simulink model "MPC_with_PI"  (R2021b)
settings: Solver=VariableStepAuto  StartTime=0.0  StopTime=115  FixedStep=0.1  RelTol=1e-2
InitFcn:
  | clear all;
  | 
  | 
  | %Path in global coordinate reference frame - X and Y
  | 
  | xRef=[
  | 57.222
  | 52.707
  | 48.874
  | 44.359
  | 39.930
  | 35.160
  | 31.071
  | 16.591
  | 7.391
  | -2.575
  | -9.901
  | -13.563
  | -16.289
  | -17.567
  | -15.437
  | -8.538
  | -2.745
  | 1.002
  | 6.624
  | 10.628
  | 15.654
  | 20.935
  | 24.853
  | 28.260
  | 31.327
  | 33.797
  | 35.841
  | 36.182
  | 35.671
  | 34.478
  | 32.008
  | 29.964
  | 28.005
  | 26.301
  | 25.109
  | 24.001
  | 23.149
  | 22.383
  | 21.957
  | 21.531
  | 21.190
  | 20.850
  | 20.594
  | 21.105
  | 21.531
  | 21.701
  | 21.701
  | 21.531
  | 21.361
  | 21.446
  | 22.042
  | 23.831
  | 25.875
  | 28.771
  | 35.245
  | 41.208
  | 49.130
  | 53.814
  | 58.585
  | 64.377
  | 71.021
  | 79.113
  | 86.439
  | 94.360
  | 100.153
  | 103.304
  | 105.400
  | 105.989
  | 105.989
  | 105.989
  | 105.989
  | 105.989
  | 106.540
  | 107.393
  | 107.904
  | 108.500
  | 109.267
  | 109.948
  | 110.204
  | 110.204
  | 110.204
  | 110.289
  | 110.204
  | 110.204
  | 110.034
  | 109.608
  | 108.500
  | 107.393
  | 106.456
  | 105.775
  | 105.775
  | 105.689
  | 105.689
  | 105.775
  | 105.689
  | 105.775
  | 105.775
  | 105.604];
  | 
  | 
  | yRef=[65.95708466
  | 66.72370911
  | 67.31997681
  | 68.17178345
  | 68.9384079
  | 69.79021454
  | 70.55683899
  | 72.43080902
  | 73.1974411
  | 73.02707672
  | 70.98274231
  | 69.44949341
  | 67.06443787
  | 63.40166855
  | 57.3538475
  | 52.15782928
  | 45.76928711
  | 39.21038055
  | 32.82183456
  | 29.92569351
  | 27.71099854
  | 26.09256744
  | 24.38895607
  | 22.42980194
  | 19.27812004
  | 16.21161842
  | 11.95258808
  | 7.182474136
  | 2.412360907
  | -1.676307797
  | -5.679795742
  | -9.257381439
  | -12.74978542
  | -16.66809273
  | -19.81977463
  | -23.05663872
  | -26.37868118
  | -30.21180725
  | -33.53385162
  | -36.855896
  | -40.34830093
  | -43.75552368
  | -49.03672028
  | -58.32140732
  | -65.81729889
  | -81.49052429
  | -89.32714081
  | -106.0225372
  | -109.0890427
  | -111.8148193
  | -114.6257782
  | -116.2
  | -116.4997559
  | -116.4997559
  | -116.4997559
  | -116.4997559
  | -116.4997559
  | -116.4997559
  | -116.4997559
  | -116.4997559
  | -116.4997559
  | -116.4997559
  | -116.0738525
  | -116.0738525
  | -116.0738525
  | -115.7331314
  | -114.7961426
  | -113.1777115
  | -110.7074738
  | -106.7039871
  | -99.20809174
  | -92.47882843
  | -87.19763184
  | -85.40883636
  | -83.70522308
  | -82.17197418
  | -80.63872528
  | -78.25366211
  | -75.35752869
  | -71.86511993
  | -63.94332504
  | -56.95851517
  | -51.16623688
  | -45.20359421
  | -42.90371704
  | -40.26311874
  | -37.62252045
  | -35.2374649
  | -33.19313049
  | -30.63771057
  | -27.91193199
  | -25.35651398
  | -19.73459435
  | -13.51641083
  | -7.29822731
  | -1.505946636
  | 3.775250435
  | 19.87438393];
  | 
  | %initial positions for the car
  | X_o=57.22167206;
  | Y_o=65.95708466;
  | psi_o=2.971793445;
  | 
  | %Useless code, used for plotter XY block.
  | s = size(xRef);
  | Ts=str2double(get_param(gcs, 'StopTime'));
  | tRef = (linspace(0,Ts,s(1)))';
libraries: autolibutils x4, autolibshared x2, sim3dlib x2, vehdynlibviscommon x1, slpidlib x1, simulink x1, vdynlib x1, vehdynlibsteering x1, eeGeneralControl x1, dspvision x1
(part 1 of 3)
settings Model: Creator=tapan  LastModifiedBy=tapan
settings SolverCC: ZeroCrossAlgorithm=Adaptive

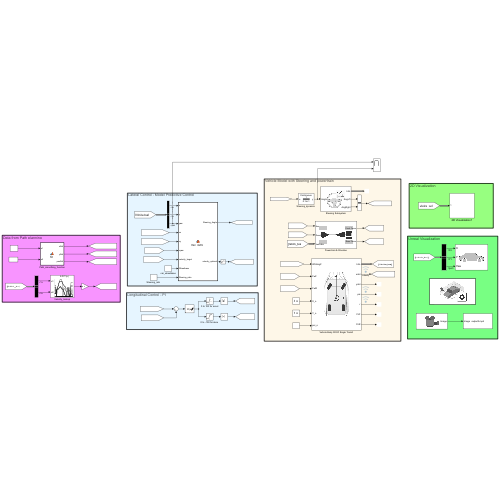
[thumbnail: Simulink's stored preview of the top-level diagram]
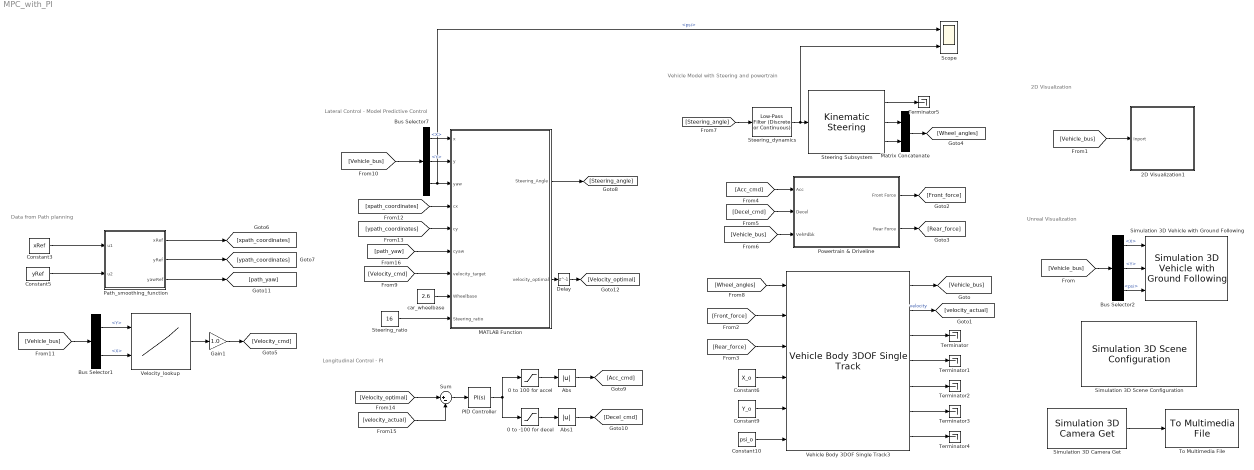
== system MPC_with_PI ==
  note: Data from Path planning
  note: Longitudinal Control - PI
  note: Vehicle Model with Steering and powertrain
  note: Unreal Visualization
  note: 2D Visualization
  note: Lateral Control - Model Predictive Control
  0 to -100 for decel : Saturate  UpperLimit=0  LowerLimit=-100
  0 to 100 for accel : Saturate  UpperLimit=100  LowerLimit=0
  2D Visualization1 : Subsystem
  Abs : Abs
  Abs1 : Abs
  Bus Selector1 : BusSelector  OutputSignals=InertFrm.Cg.Disp.Y,InertFrm.Cg.Disp.X
  Bus Selector2 : BusSelector  OutputSignals=InertFrm.Cg.Disp.X,InertFrm.Cg.Disp.Y,InertFrm.Cg.Ang.psi
  Bus Selector7 : BusSelector  OutputSignals=InertFrm.Cg.Disp.X,InertFrm.Cg.Disp.Y,InertFrm.Cg.Ang.psi
  Constant10 : Constant  Value=psi_o
  Constant3 : Constant  Value=xRef  SampleTime=0.1
  Constant5 : Constant  Value=yRef  SampleTime=0.1
  Constant6 : Constant  Value=X_o
  Constant9 : Constant  Value=Y_o
  Delay : Delay  DelayLength=1  InitialCondition=0
  Gain1 : Gain  Gain=1.0
  MATLAB Function : MATLAB Function
  Matrix Concatenate : Concatenate
  PID Controller : slpidlib/PID Controller  Controller=PI  Form=Parallel  TimeDomain=Continuous-time  UseExternalTs=off  SampleTime=-1  IntegratorMethod=Forward Euler  FilterMethod=Forward Euler  ControllerParametersSource=internal  P=1  I=5  D=0  UseFilter=on  N=100  TunerSelectOption=Transfer Function Based (PID Tuner App)  InitialConditionSource=internal  InitialConditionForIntegrator=0  InitialConditionForFilter=0  DifferentiatorICPrevScaledInput=0  ExternalReset=none  TrackingMode=off  Kt=1  LimitOutput=on  SatLimitsSource=internal  UpperSaturationLimit=100  LowerSaturationLimit=-100  LinearizeAsGain=on  AntiWindupMode=clamping  Kb=1  POutMin=[]  POutMax=[]  IOutMin=[]  IOutMax=[]  DOutMin=[]  DOutMax=[]  NOutMin=[]  NOutMax=[]  SumOutMin=[]  SumOutMax=[]  SaturationOutMin=[]  SaturationOutMax=[]  PParamMin=[]  PParamMax=[]  IParamMin=[]  IParamMax=[]  DParamMin=[]  DParamMax=[]  NParamMin=[]  NParamMax=[]  KbParamMin=[]  KbParamMax=[]  KtParamMin=[]  KtParamMax=[]  KbOutMin=[]  KbOutMax=[]  KtOutMin=[]  KtOutMax=[]  IntegratorOutMin=[]  IntegratorOutMax=[]  FilterOutMin=[]  FilterOutMax=[]  SumI1OutMin=[]  SumI1OutMax=[]  SumI2OutMin=[]  SumI2OutMax=[]  SumI3OutMin=[]  SumI3OutMax=[]  SumI4OutMin=[]  SumI4OutMax=[]  SumDOutMin=[]  SumDOutMax=[]  DifferentiatorOutMin=[]  DifferentiatorOutMax=[]  FilterDiffOutCoefMin=[]  FilterDiffOutCoefMax=[]  ReciprocalOutMin=[]  ReciprocalOutMax=[]  SumDenOutMin=[]  SumDenOutMax=[]  SumNumOutMin=[]  SumNumOutMax=[]  DivideOutMin=[]  DivideOutMax=[]  UdiffTsProdOutMin=[]  UdiffTsProdOutMax=[]  NTsProdOutMin=[]  NTsProdOutMax=[]  UintegralTsProdOutMin=[]  UintegralTsProdOutMax=[]  UngainTsProdOutMin=[]  UngainTsProdOutMax=[]  IntegratorContinuousStateAttributes=''  IntegratorStateMustResolveToSignalObject=off  IntegratorRTWStateStorageClass=Auto  FilterContinuousStateAttributes=''  FilterStateMustResolveToSignalObject=off  FilterRTWStateStorageClass=Auto  ParallelPVariant=InternalParameters  IdealPVariant=Disabled  IVariant=InternalParameters  DVariant=Disabled  IntegratorVariant=Continuous  SatVariant=Enabled  AWVariant=ContClampingParallel  PCopyVariant=Disabled  TRVariant=Disabled  FdbkBlocksVariant=Forward  IdealPFdbkVariant=Disabled  SatFdbkVariant=Disabled  DerivativeFilterVariant=Disabled  NVariant=Disabled  NCopyVariant=Disabled_SignalSpec  FilterICVariant=Disabled  IntegratorICVariant=InternalICs  ExternalResetVariant=Disabled  TRSumVariant=Passthrough  SumFdbkVariant=Disabled  SumVariant=Sum_PI  TsampFilterVariant=InternalTs  TsampNgainVariant=Passthrough  TsampIntegralVariant=Passthrough  ExternalSaturationOutDataTypeStr=Inherit: Same as second input
  Path_smoothing_function : MATLAB Function  TreatAsAtomicUnit=on
  Powertrain & Driveline : Subsystem
      mask Display: image('vdbslibpt.png');
  Scope : Scope  NumInputPorts=2
  Simulation 3D Camera Get : sim3dlib/Simulation 3D Camera Get  Priority=1  sensorTag=Sim3dSensor1  sensorId=1  sensorName=Sim3dSensor1  vehTagList={'Scene Origin';'SimulinkVehicle1'}  vehTag=SimulinkVehicle1  mountLoc=Hood center  offsetFlag=on  tmountOffset=[-10, 0, 7]  rmountOffset=[0, 25, 0]  HorizontalResolution=1280  VerticalResolution=720  HorizontalFOV=120  SampleTime=-1  mountPoint=[-8.53600025177002 0 8.10000038146973]  mountOrientation=[0 -25 0]  aMode=2  ID=1
      settings: SourceProductBaseCode=AE,DR,UV,VE
  Simulation 3D Scene Configuration : sim3dlib/Simulation 3D Scene Configuration  Priority=0  ProjectFormat_internal=Default Scenes  ProjectFormat=Default Scenes  SceneDesc=Virtual Mcity  ProjectName=C:\Program Files\MATLAB\R2021b\toolbox\shared\sim3d_projects\automotive_project\UE4\WindowsNoEditor\VehicleSimulation.exe  ScenePath=/Game/Maps/HwStrght  vehTagList={'Scene Origin';'SimulinkVehicle1'}  vehTag=SimulinkVehicle1  OpVisEn=off  Ts=0.05  EnableWindow=off  EnableWeather=off  SunAltitude=40.0  SunAzimuth=90  clouds=10  wind=1  fog=0  rain=0  sensorTag=MainCamera1  sensorId=1  sensorName=MainCamera1  mountLoc=Origin  offsetFlag=off  tmountOffset=[0, 0, 0]  rmountOffset=[0, 0, 0]  HorizontalResolution=1280  VerticalResolution=720  HorizontalFOV=60  mountPoint=[0 0 0]  mountOrientation=[0 0 0]  aMode=3  ID=1
      settings: SourceProductBaseCode=AE,DR,UV,VE
  Simulation 3D Vehicle with Ground Following : vdynlib/Vehicle Scenarios/Sim3D/Sim3D Vehicle/Components/Simulation 3D Vehicle with Ground Following  Priority=-1  PassVehMesh=Sedan  PassVehMesh_Internal=Sedan  MeshPath=/MathWorksSimulation/Vehicles/Muscle/Meshes/SK_MuscleCar.SK_MuscleCar  TrackWidth=1.9  WheelBase=3  WheelRadius=0.35  VehColor=Silver  VehColor_Internal=Silver  InitialPos=[0, 0, 0]  InitialRot=[0, 0, 0]  ActorName=SimulinkVehicle1  VehLightsControl=off  HeadlightColor=[ 1, 1, 1 ]  HighBeamIntensity=100000  LowBeamIntensity=60000  HighBeamConeAngle=1.22  LowBeamConeAngle=1.22  LeftHeadlightOrientation=[ 0, 0 ]  RightHeadlightOrientation=[ 0, 0 ]  BrakelightIntensity=200  ReverselightIntensity=500  SignallightIntensity=500  SignallightPeriod=1  SignalPulseWidth=50  SampleTime=-1  ActorType=SimulinkVehicle  ID=1  aMode=2  ActorTag=SimulinkVehicle1  CoordinateScheme=SAE
      settings: SourceProductBaseCode=VE
  Steering Subsystem : vehdynlibsteering/Kinematic Steering  StrgType=Ackerman  StrgRatioType=Constant  Loc=Front  NrmlFctr=0.01  TrckWdth=1.4  WhlBase=2.6  Db=0  StrgRng=5*pi  StrgAngBpts="[-6.2832   -5.0265   -3.7699   -2.5133   -1.2566         0    1.2566    2.5133    3.7699    5.0265    6.2832]"  StrgRatioTbl=|  StrgRatio=16  StrgArmLngth=0.1  RckCsLngth=0.5  TieRodLngth=0.248  D=0.2  PnnRadius=0.0057  PnnRadiusTbl="[0.0055    0.0055    0.0056    0.0057    0.0058    0.0057    0.0057    0.0057    0.0056    0.0055    0.0055]"  RodLngth=0.1  ParaArmLngth=0.9  aMode=2
      | [13.5000   13.3750   13.2500   13.1250   13.0000   13.0000   13.0000   13.1250   13.2500   13.3750   13.5000
      | ]
  Steering_dynamics : eeGeneralControl/Low-Pass Filter (Discrete or Continuous)  K=1  T=0.1  B=inf  A=-inf  init_option=Inherited from block input  x0=0  Ts=0
  Steering_ratio : Constant  Value=16
  Sum : Sum  Inputs=|+-
  Terminator{,1..5} (6 alike) : Terminator
  To Multimedia File : dspvision/To Multimedia File  outputFilename=C:\Users\tapan\Desktop\output2.mp4  streamSelection=Video only  videoCompressor=None (uncompressed)  audioCompressor=None (uncompressed)  imagePorts=One multidimensional signal  fileType=MPEG4  audioDatatype=Determine from input data type  fourcc=RGB  videoQuality=75  mj2000CompFactor=10
  Vehicle Body 3DOF Single Track3 : autolibshared/Vehicle Body 3DOF Single Track  trackMode=Dual  inputMode=External longitudinal forces  frontSteerMode=on  rearSteerMode=off  windMode=off  muMode=off  extFMode=off  extMMode=off  htchFMode=off  htchMMode=off  extXo=on  extpsio=on  extxdoto=off  extro=off  extYo=on  extTamb=off  extydoto=off  aMode=2  NF=2  NR=2  m=1625  a=1.135  b=1.465  h=0.509  dh=1  hh=0.2  X_o=0  xdot_o=1  CalphaMode=off  sigmaMode=off  d=0  hl=0  w=[1.4,1.4]  Cy_f=12e3  Cy_r=11e3  sigma_f=.1  sigma_r=.1  alpha_f_brk=[-.1 .1]  Cy_f_data=[-9e3 9e3]  alpha_r_brk=[-.1 .1]  Cy_r_data=[-9e3 9e3]  Y_o=0  ydot_o=0  Izz=2045  psi_o=0  r_o=0  Af=2  Cd=.3  Cl=.1  Cpm=.1  beta_w=[0:0.01:0.3]  Cs=[0:0.03:0.9]  Cym=[0:0.01:0.3]  Pabs=101325  Tair=273  g=9.81  mu=1  xdot_tol=.01  Fznom=5000  Fxtire_sat=7e4  Fytire_sat=7e4  longOff=0  latOff=0  vertOff=0  wrapAng=off
      settings: SourceProductBaseCode=PW,DR,MT,UV,VE
  Velocity_lookup : Lookup_n-D  BreakpointsForDimension1=|  BreakpointsForDimension2="[-20\t-10\t0\t10\t20\t30\t40\t50\t60\t70\t80\t90\t100\t110\t120]"  Table=|  InternalRulePriority=Speed  RndMeth=Simplest  InputSameDT=on
      BreakpointsForDimension1=|
      | [-120
      | -110
      | -100
      | -90
      | -80
      | -70
      | -60
      | -50
      | -40
      | -30
      | -20
      | -10
      | 0
      | 10
      | 20
      | 30
      | 40
      | 50
      | 60
      | 70
      | 80]
      Table=|
      | [0	0	0	2	2	2	4	5.60000000000000	7.20000000000000	5.60000000000000	4.80000000000000	3.50000000000000	2	2	0
      | 0	0	0	2	2	2	4	5.60000000000000	7.20000000000000	5.60000000000000	4.80000000000000	3.50000000000000	2	2	0
      | 0	0	0	4	4	4	0	0	0	0	0	0	4	4	0
      | 0	0	0	5.60000000000000	5.60000000000000	5.60000000000000	0	0	0	0	0	0	4.80000000000000	4.80000000000000	4.80000000000000
      | 0	0	0	7.20000000000000	7.20000000000000	7.20000000000000	0	0	0	0	0	0	4.80000000000000	4.80000000000000	4.80000000000000
      | 0	0	0	9.50000000000000	9.50000000000000	9.50000000000000	0	0	0	0	0	0	5.60000000000000	5.60000000000000	5.60000000000000
      | 0	0	0	9.50000000000000	11	9.50000000000000	0	0	0	0	0	0	6.40000000000000	6.40000000000000	6.40000000000000
      | 0	0	0	9.50000000000000	11	9.50000000000000	0	0	0	0	0	0	5.60000000000000	5.60000000000000	5.60000000000000
      | 0	0	0	9.50000000000000	9.50000000000000	9.50000000000000	0	0	0	0	0	0	4.80000000000000	4.80000000000000	4.80000000000000
      | 0	0	0	0	8	8	0	0	0	0	0	0	4.80000000000000	4.80000000000000	4.80000000000000
      | 0	0	0	0	7.20000000000000	7.20000000000000	5.60000000000000	0	0	0	0	0	3.20000000000000	3.20000000000000	3.20000000000000
      | 0	0	0	0	6.40000000000000	6.40000000000000	4.80000000000000	0	0	0	0	0	1.60000000000000	1.60000000000000	1.60000000000000
      | 0	0	0	0	6.40000000000000	5.60000000000000	4	0	0	0	0	0	0	0	0
      | 0	0	0	0	0	4.80000000000000	3.20000000000000	0	0	0	0	0	0	0	0
      | 0	0	0	5.60000000000000	5.60000000000000	4.80000000000000	3.20000000000000	0	0	0	0	0	0	0	0
      | 0	0	5.60000000000000	4.80000000000000	5.60000000000000	4.80000000000000	4	0	0	0	0	0	0	0	0
      | 0	4	5.60000000000000	4.80000000000000	0	0	0	0	0	0	0	0	0	0	0
      | 2.40000000000000	3.20000000000000	4.80000000000000	0	0	0	0	0	1.60000000000000	1.60000000000000	0	0	0	0	0
      | 2.40000000000000	3.20000000000000	4.80000000000000	7.20000000000000	8.80000000000000	6.40000000000000	4	1.60000000000000	1.60000000000000	1.60000000000000	0	0	0	0	0
      | 2.40000000000000	3.20000000000000	4.80000000000000	7.20000000000000	8.80000000000000	6.40000000000000	4	1.60000000000000	1.60000000000000	1.60000000000000	0	0	0	0	0
      | 2.40000000000000	3.20000000000000	4.80000000000000	7.20000000000000	8.80000000000000	6.40000000000000	4	1.60000000000000	0	0	0	0	0	0	0]
      settings: InputPortMap=u0,u1
  car_wheelbase : Constant  Value=2.6
  wires:
  Constant10/1 -> Vehicle Body 3DOF Single Track3/6
  Constant9/1 -> Vehicle Body 3DOF Single Track3/5
  Constant6/1 -> Vehicle Body 3DOF Single Track3/4
  Constant3/1 -> Path_smoothing_function/1(u1)
  Constant5/1 -> Path_smoothing_function/2(u2)
  Bus Selector2/2 -> Simulation 3D Vehicle with Ground Following/2  "<Y>"
  Bus Selector2/1 -> Simulation 3D Vehicle with Ground Following/1  "<X>"
  Bus Selector2/3 -> Simulation 3D Vehicle with Ground Following/3  "<psi>"
  Steering Subsystem/2 -> Matrix Concatenate/1
  Steering Subsystem/3 -> Matrix Concatenate/2
  PID Controller/1 -> 0 to -100 for decel/1, 0 to 100 for accel/1
  Sum/1 -> PID Controller/1
  0 to 100 for accel/1 -> Abs/1
  0 to -100 for decel/1 -> Abs1/1
  Vehicle Body 3DOF Single Track3/1 -> [Vehicle_bus]
  Vehicle Body 3DOF Single Track3/2 -> [velocity_actual]  "velocity"
  [Vehicle_bus] -> Bus Selector2/1
  [Vehicle_bus] -> 2D Visualization1/1(Inport)
  Steering_dynamics/1 -> Scope/2, Steering Subsystem/1
  Vehicle Body 3DOF Single Track3/3 -> Terminator/1
  Vehicle Body 3DOF Single Track3/4 -> Terminator1/1
  Vehicle Body 3DOF Single Track3/5 -> Terminator2/1
  Vehicle Body 3DOF Single Track3/6 -> Terminator3/1
  Vehicle Body 3DOF Single Track3/7 -> Terminator4/1
  Powertrain & Driveline/1(Front Force) -> [Front_force]
  Powertrain & Driveline/2(Rear Force) -> [Rear_force]
  [Acc_cmd] -> Powertrain & Driveline/1(Acc)
  [Decel_cmd] -> Powertrain & Driveline/2(Decel)
  [Vehicle_bus] -> Powertrain & Driveline/3(VehFdbk)
  Matrix Concatenate/1 -> [Wheel_angles]
  [Steering_angle] -> Steering_dynamics/1
  [Wheel_angles] -> Vehicle Body 3DOF Single Track3/1
  Bus Selector1/2 -> Velocity_lookup/2  "<X>"
  Bus Selector1/1 -> Velocity_lookup/1  "<Y>"
  Path_smoothing_function/1(xRef) -> [xpath_coordinates]
  Path_smoothing_function/2(yRef) -> [ypath_coordinates]
  [Vehicle_bus] -> Bus Selector1/1
  Abs1/1 -> [Decel_cmd]
  Abs/1 -> [Acc_cmd]
  [Velocity_optimal] -> Sum/1
  [velocity_actual] -> Sum/2
  Steering Subsystem/1 -> Terminator5/1
  Path_smoothing_function/3(yawRef) -> [path_yaw]
  Velocity_lookup/1 -> Gain1/1
  [Velocity_cmd] -> MATLAB Function/7(velocity_target)
  MATLAB Function/1(Steering_Angle) -> [Steering_angle]
  [ypath_coordinates] -> MATLAB Function/5(cy)
  Bus Selector7/3 -> MATLAB Function/3(yaw), Scope/1  "<psi>"
  Bus Selector7/1 -> MATLAB Function/1(x)  "<X>"
  [xpath_coordinates] -> MATLAB Function/4(cx)
  [path_yaw] -> MATLAB Function/6(cyaw)
  Bus Selector7/2 -> MATLAB Function/2(y)  "<Y>"
  [Vehicle_bus] -> Bus Selector7/1
  car_wheelbase/1 -> MATLAB Function/8(Wheelbase)
  Gain1/1 -> [Velocity_cmd]
  Simulation 3D Camera Get/1 -> To Multimedia File/1
  Steering_ratio/1 -> MATLAB Function/9(Steering_ratio)
  MATLAB Function/2(velocity_optimal) -> Delay/1
  Delay/1 -> [Velocity_optimal]
  [Front_force] -> Vehicle Body 3DOF Single Track3/2
  [Rear_force] -> Vehicle Body 3DOF Single Track3/3

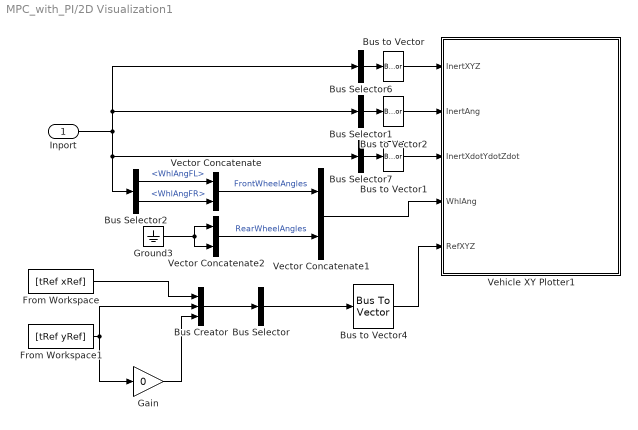
== system MPC_with_PI/2D Visualization1 ==
  Inport : Inport
  Bus Creator : BusCreator  Inputs=3
  Bus Selector : BusSelector  OutputSignals=signal1,signal2,signal3  OutputAsBus=on
  Bus Selector1 : BusSelector  OutputSignals=InertFrm.Cg.Ang.phi,InertFrm.Cg.Ang.theta,InertFrm.Cg.Ang.psi  OutputAsBus=on
  Bus Selector2 : BusSelector  OutputSignals=BdyFrm.FrntAxl.Steer.WhlAngFL,BdyFrm.FrntAxl.Steer.WhlAngFR
  Bus Selector6 : BusSelector  OutputSignals=InertFrm.Geom.Disp.X,InertFrm.Geom.Disp.Y,InertFrm.Geom.Disp.Z  OutputAsBus=on
  Bus Selector7 : BusSelector  OutputSignals=InertFrm.Geom.Vel.Xdot,InertFrm.Geom.Vel.Ydot,InertFrm.Geom.Vel.Zdot  OutputAsBus=on
  Bus to Vector{,1..2,4} (4 alike) : BusToVector
  From Workspace : FromWorkspace  VariableName=[tRef xRef]
  From Workspace1 : FromWorkspace  VariableName=[tRef yRef]
  Gain : Gain  Gain=0
  Ground3 : Ground
  Vector Concatenate : Concatenate
  Vector Concatenate1 : Concatenate
  Vector Concatenate2 : Concatenate
  Vehicle XY Plotter1 : Subsystem  mask(Vehicle XY Plotter){extRef=on, extStats=off, extTireF=off, a=1.135, b=1.465, w=1.4, figBorder=15, bufferSize=1024, velNorm=10, tireFNorm=1000, pltDT=0.5}
      mask prompts: extRef "Plot path reference, extRef"; extStats "Display speed, RPM and Gear"; extTireF "Display tire forces"; a "Distance to front axle from CG, a [m]:"; b "Distance to rear axle from CG, b [m]:"; w "Track width, w [m]:"; figBorder "Distance to figure borders, figBorder [m]:"; bufferSize "Path buffer sampe size, bufferSize []:"; velNorm "Velocity vector scaling, velNorm [m*s/m]:"; tireFNorm "Tire force vector scaling, tireFNorm [m/N]:"; pltDT "Plot update rate, pltDT [s]:"
      mask help:
      | This block will display a MATLAB figure which indicates the vehicle path, current position and heading velocity.
      | An optional path reference is also provided.
      mask init:
      | block = gcb;
      | if autoblkschecksimstopped(block)
      |     ParamNames = {'extRef';'extStats';'extTireF';'extTireF'};
      |     PortNames = {'RefXYZ';'Stats';'TireFx';'TireFy'};
      |     for idx=1:length(PortNames)
      |         InportOption  = {'built-in/Ground', [PortNames{idx}, ' Ground'];...
      |             'built-in/Inport',PortNames{idx}};
      |         if ~strcmp(get_param(block,ParamNames{idx}),'on')
      |             NewBlkHdl = autoblksreplaceblock(block, InportOption, 1);
      |             set_param(NewBlkHdl, 'ShowName', 'off');
      |         else
      |             autoblksreplaceblock(block, InportOption, 2);
      |         end
      |     end
      |     InportNames = {'InertXYZ';'InertAng';'InertXdotYdotZdot';'WhlAng';'RefXYZ';'Stats';'TireFx';'TireFy'};
      |     FoundNames = get_param(find_system(block, 'LookUnderMasks', 'all', 'SearchDepth', 1, 'FollowLinks', 'on', 'BlockType', 'Inport'), 'Name');
      |     [~,PortI] = intersect(InportNames, FoundNames);
      |     PortI = sort(PortI);
      |     for idx = 1:length(PortI)
      |         set_param([block, '/', InportNames{PortI(idx)}], 'Port', num2str(idx));
      |     end
      | end
      mask TypeOptions a: Vehicle XY Plotter/a
      mask TypeOptions b: Vehicle XY Plotter/b
      mask TypeOptions w: Vehicle XY Plotter/w
      mask TypeOptions figBorder: Vehicle XY Plotter/figBorder
      mask TypeOptions bufferSize: Vehicle XY Plotter/bufferSize
      mask TypeOptions velNorm: Vehicle XY Plotter/velNorm
      mask TypeOptions tireFNorm: Vehicle XY Plotter/tireFNorm
      mask DialogControl Container3 Prompt: Plot and Display Options
  wires:
  Bus Creator/1 -> Bus Selector/1
  From Workspace/1 -> Bus Creator/1
  Gain/1 -> Bus Creator/3
  From Workspace1/1 -> Bus Creator/2, Gain/1
  Bus Selector/1 -> Bus to Vector4/1
  Bus to Vector4/1 -> Vehicle XY Plotter1/5(RefXYZ)
  Inport/1 -> Bus Selector6/1, Bus Selector1/1, Bus Selector2/1, Bus Selector7/1
  Bus Selector2/2 -> Vector Concatenate/2  "<WhlAngFR>"
  Bus Selector1/1 -> Bus to Vector2/1
  Bus to Vector2/1 -> Vehicle XY Plotter1/2(InertAng)
  Bus to Vector/1 -> Vehicle XY Plotter1/1(InertXYZ)
  Bus to Vector1/1 -> Vehicle XY Plotter1/3(InertXdotYdotZdot)
  Bus Selector7/1 -> Bus to Vector1/1
  Vector Concatenate2/1 -> Vector Concatenate1/2  "RearWheelAngles"
  Bus Selector2/1 -> Vector Concatenate/1  "<WhlAngFL>"
  Vector Concatenate/1 -> Vector Concatenate1/1  "FrontWheelAngles"
  Bus Selector6/1 -> Bus to Vector/1
  Ground3/1 -> Vector Concatenate2/2, Vector Concatenate2/1
  Vector Concatenate1/1 -> Vehicle XY Plotter1/4(WhlAng)

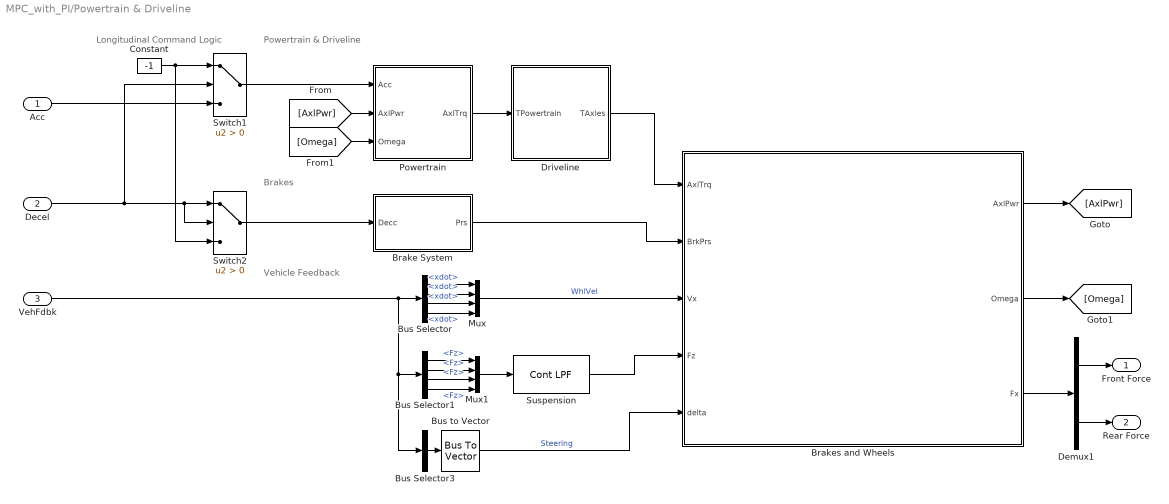
== system MPC_with_PI/Powertrain & Driveline ==
  note: Vehicle Feedback
  note: Powertrain & Driveline
  note: Brakes
  note: Longitudinal Command Logic
  Acc : Inport
  Decel : Inport  Port=2
  VehFdbk : Inport  Port=3
  Brake System : Subsystem
  Brakes and Wheels : Subsystem  TreatAsAtomicUnit=on
      mask Display: image('vdbslibwhls.png');
  Bus Selector : BusSelector  OutputSignals=BdyFrm.FrntAxl.Lft.Vel.xdot,BdyFrm.FrntAxl.Rght.Vel.xdot,BdyFrm.RearAxl.Lft.Vel.xdot,BdyFrm.RearAxl.Rght.Vel.xdot
  Bus Selector1 : BusSelector  OutputSignals=BdyFrm.Forces.FrntAxl.Lft.Fz,BdyFrm.Forces.FrntAxl.Rght.Fz,BdyFrm.Forces.RearAxl.Lft.Fz,BdyFrm.Forces.RearAxl.Rght.Fz
  Bus Selector3 : BusSelector  OutputSignals=BdyFrm.FrntAxl.Steer.WhlAngFL,BdyFrm.FrntAxl.Steer.WhlAngFR,BdyFrm.RearAxl.Steer.WhlAngRL,BdyFrm.RearAxl.Steer.WhlAngRR  OutputAsBus=on
  Bus to Vector : BusToVector
  Constant : Constant  Value=-1
  Demux1 : Demux  Outputs=[2 2]
  Driveline : Subsystem  Variant=on  VariantControlMode=label  VariantControl=Variant1  LabelModeActiveChoice=1
  Mux : Mux
  Mux1 : Mux
  Powertrain : Subsystem
  Suspension : autolibutils/Cont LPF  wc=10*pi*2  aMode=2
      settings: SourceProductBaseCode=PW,DR,MT,UV,VE
  Switch1 : Switch  Criteria=u2 > Threshold
  Switch2 : Switch  Criteria=u2 > Threshold
  Front Force : Outport  VectorParamsAs1DForOutWhenUnconnected=off
  Rear Force : Outport  Port=2  VectorParamsAs1DForOutWhenUnconnected=off
  wires:
  Brake System/1(Prs) -> Brakes and Wheels/2(BrkPrs)
  Switch2/1 -> Brake System/1(Decc)
  [Omega] -> Powertrain/3(Omega)
  [AxlPwr] -> Powertrain/2(AxlPwr)
  Brakes and Wheels/2(Omega) -> [Omega]
  Powertrain/1(AxlTrq) -> Driveline/1(TPowertrain)
  Switch1/1 -> Powertrain/1(Acc)
  Bus Selector1/4 -> Mux1/4  "<Fz>"
  Bus Selector1/3 -> Mux1/3  "<Fz>"
  Bus Selector1/2 -> Mux1/2  "<Fz>"
  Bus Selector1/1 -> Mux1/1  "<Fz>"
  Bus Selector/4 -> Mux/4  "<xdot>"
  Bus Selector/3 -> Mux/3  "<xdot>"
  Bus Selector/2 -> Mux/2  "<xdot>"
  Bus Selector/1 -> Mux/1  "<xdot>"
  Suspension/1 -> Brakes and Wheels/4(Fz)
  Mux1/1 -> Suspension/1
  Bus to Vector/1 -> Brakes and Wheels/5(delta)  "Steering"
  Bus Selector3/1 -> Bus to Vector/1
  Brakes and Wheels/3(Fx) -> Demux1/1
  Brakes and Wheels/1(AxlPwr) -> [AxlPwr]
  Driveline/1(TAxles) -> Brakes and Wheels/1(AxlTrq)
  Demux1/2 -> Rear Force/1
  Demux1/1 -> Front Force/1
  VehFdbk/1 -> Bus Selector/1, Bus Selector1/1, Bus Selector3/1
  Mux/1 -> Brakes and Wheels/3(Vx)  "WhlVel"
  Constant/1 -> Switch1/1, Switch2/3
  Acc/1 -> Switch1/3
  Decel/1 -> Switch2/1, Switch2/2, Switch1/2

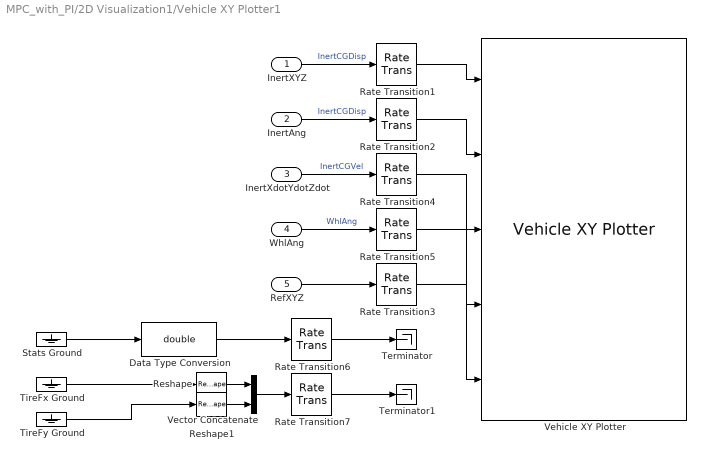
== system MPC_with_PI/2D Visualization1/Vehicle XY Plotter1 ==
  InertXYZ : Inport
  InertAng : Inport  Port=2
  InertXdotYdotZdot : Inport  Port=3
  WhlAng : Inport  Port=4
  RefXYZ : Inport  Port=5
  Data Type Conversion : DataTypeConversion  OutDataTypeStr=double
  Rate Transition{1..7} (7 alike) : RateTransition  Deterministic=off  OutPortSampleTime=pltDT
  Reshape : Reshape  OutputDimensionality=Row vector (2-D)
  Reshape1 : Reshape  OutputDimensionality=Row vector (2-D)
  Stats Ground : Ground
  Terminator : Terminator
  Terminator1 : Terminator
  TireFx Ground : Ground
  TireFy Ground : Ground
  Vector Concatenate : Concatenate  Mode=Multidimensional array
  Vehicle XY Plotter : vehdynlibviscommon/Vehicle XY Plotter  w=w  a=a  b=b  figBorder=figBorder  bufferSize=bufferSize  extStats=off  extTireF=off
      settings: SourceProductBaseCode=VE
  wires:
  TireFy Ground/1 -> Reshape1/1
  TireFx Ground/1 -> Reshape/1
  Stats Ground/1 -> Data Type Conversion/1
  InertAng/1 -> Rate Transition2/1  "InertCGDisp"
  InertXdotYdotZdot/1 -> Rate Transition4/1  "InertCGVel"
  InertXYZ/1 -> Rate Transition1/1  "InertCGDisp"
  WhlAng/1 -> Rate Transition5/1  "WhlAng"
  Rate Transition3/1 -> Vehicle XY Plotter/5
  Rate Transition1/1 -> Vehicle XY Plotter/1
  Rate Transition2/1 -> Vehicle XY Plotter/2
  Rate Transition4/1 -> Vehicle XY Plotter/3
  Rate Transition5/1 -> Vehicle XY Plotter/4
  Rate Transition6/1 -> Terminator/1
  Data Type Conversion/1 -> Rate Transition6/1
  Rate Transition7/1 -> Terminator1/1
  RefXYZ/1 -> Rate Transition3/1
  Reshape/1 -> Vector Concatenate/1
  Reshape1/1 -> Vector Concatenate/2
  Vector Concatenate/1 -> Rate Transition7/1

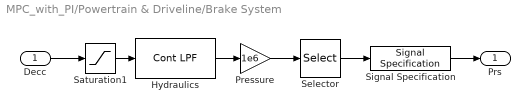
== system MPC_with_PI/Powertrain & Driveline/Brake System ==
  Decc : Inport
  Hydraulics : autolibutils/Cont LPF  wc=30*pi*2  aMode=2
      settings: SourceProductBaseCode=PW,DR,MT,UV,VE
  Pressure : Gain  Gain=1e6
  Saturation1 : Saturate  UpperLimit=inf  LowerLimit=0  ZeroCross=off
  Selector : Selector  InputPortWidth=1  IndexOptions=Index vector (dialog)  Indices=[1 1 1 1]  OutputSizes=1
  Signal Specification : SignalSpecification  Unit=Pa
  Prs : Outport  VectorParamsAs1DForOutWhenUnconnected=off
  wires:
  Signal Specification/1 -> Prs/1
  Decc/1 -> Saturation1/1
  Selector/1 -> Signal Specification/1
  Saturation1/1 -> Hydraulics/1
  Hydraulics/1 -> Pressure/1
  Pressure/1 -> Selector/1
